simulink model "questao8_ajuste"  (R2023a)
settings: Solver=VariableStepAuto  StartTime=0.0  StopTime=160  FixedStep=1  MaxStep=0.1  RelTol=1e-3
values from neighbouring files (symbols this model uses):
  B = 0.1    [trab_controle.m]
  J = 1    [trab_controle.m]
  Km = 1/3    (= 0.333333333333)    [trab_controle.m]
  L = 0.5    [trab_controle.m]
  R = 10    [trab_controle.m]
settings Model: Creator=franz  LastModifiedBy=franz

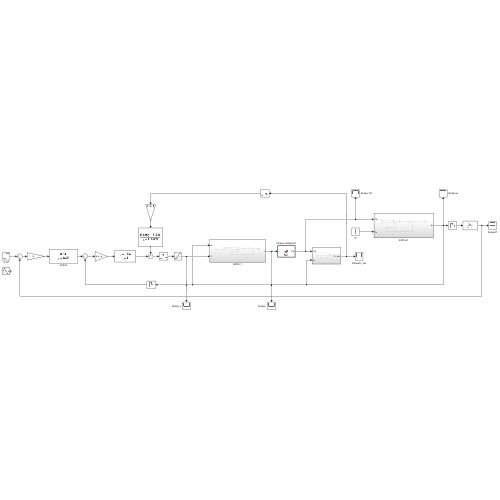
[thumbnail: Simulink's stored preview of the top-level diagram]
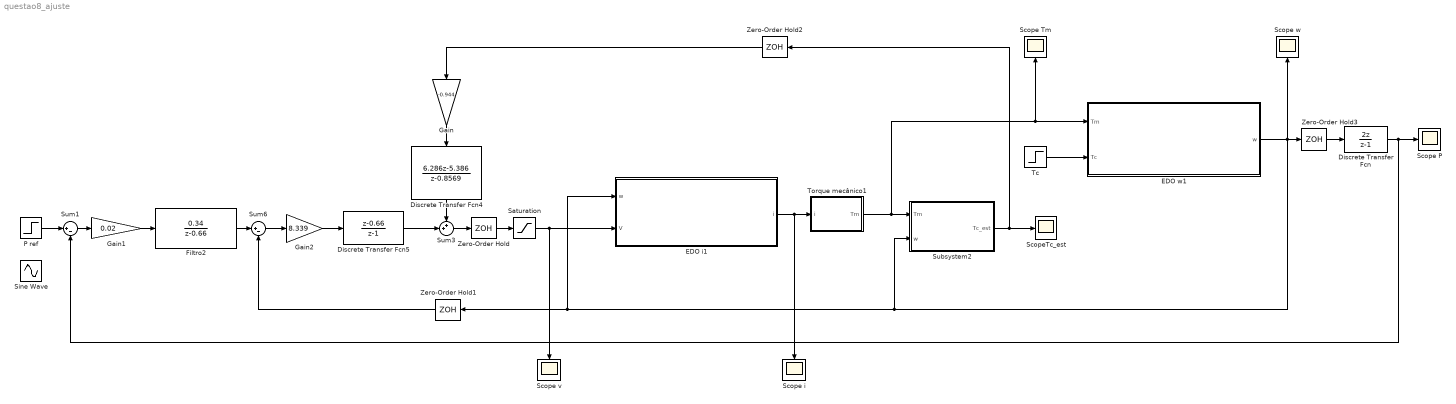
== system questao8_ajuste ==
  Discrete Transfer Fcn : DiscreteTransferFcn  Numerator=[2 0]  Denominator=[1 -1]
  Discrete Transfer Fcn4 : DiscreteTransferFcn  Numerator=[6.286 -5.386]  Denominator=[1 -0.8569]
  Discrete Transfer Fcn5 : DiscreteTransferFcn  Numerator=[1 -0.66]  Denominator=[1 -1]
  EDO i1 : Subsystem
  EDO w1 : Subsystem
  Filtro2 : DiscreteTransferFcn  Numerator=[0 0.34]  Denominator=[1 -0.66]
  Gain : Gain  Gain=-0.944
  Gain1 : Gain  Gain=0.02
  Gain2 : Gain  Gain=8.339
  P ref : Step  Time=80  After=5  SampleTime=0
  Saturation : Saturate  UpperLimit=40  LowerLimit=-40
  Scope P : Scope
  Scope Tm : Scope
  Scope i : Scope
  Scope v : Scope
  Scope w : Scope
  ScopeTc_est : Scope
  Sine Wave : Sin  Amplitude=5  Frequency=0.1  SampleTime=0
  Subsystem2 : Subsystem
  Sum1 : Sum  Inputs=|+-
  Sum3 : Sum  Inputs=++|
  Sum6 : Sum  Inputs=|+-
  Tc : Step  Time=120  Before=1.5  After=1.75  SampleTime=0
  Torque mecânico1 : MATLAB Function  TreatAsAtomicUnit=on
  Zero-Order Hold{,1..3} (4 alike) : ZeroOrderHold  SampleTime=-1
  wires:
  Discrete Transfer Fcn5/1 -> Sum3/2
  Filtro2/1 -> Sum6/1
  Discrete Transfer Fcn4/1 -> Sum3/1
  Sum6/1 -> Gain2/1
  Gain2/1 -> Discrete Transfer Fcn5/1
  Subsystem2/1(Tc_est) -> ScopeTc_est/1, Zero-Order Hold2/1
  EDO i1/1(i) -> Torque mecânico1/1(i), Scope i/1
  Torque mecânico1/1(Tm) -> Subsystem2/1(Tm), EDO w1/1(Tm), Scope Tm/1
  Tc/1 -> EDO w1/2(Tc)
  EDO w1/1(w) -> Zero-Order Hold3/1, Zero-Order Hold1/1, EDO i1/1(w), Subsystem2/2(w), Scope w/1
  Sum3/1 -> Zero-Order Hold/1
  Gain/1 -> Discrete Transfer Fcn4/1
  Zero-Order Hold/1 -> Saturation/1
  Zero-Order Hold1/1 -> Sum6/2
  Zero-Order Hold2/1 -> Gain/1
  Saturation/1 -> EDO i1/2(V), Scope v/1
  Discrete Transfer Fcn/1 -> Scope P/1, Sum1/2
  Sum1/1 -> Gain1/1
  Gain1/1 -> Filtro2/1
  Zero-Order Hold3/1 -> Discrete Transfer Fcn/1
  P ref/1 -> Sum1/1

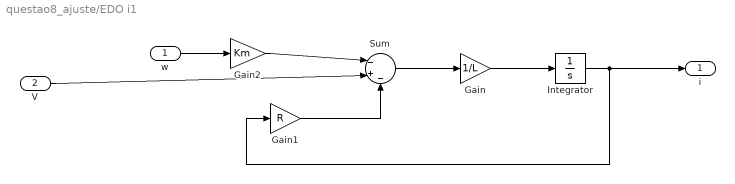
== system questao8_ajuste/EDO i1 ==
  w : Inport
  V : Inport  Port=2
  Gain : Gain  Gain=1/L
  Gain1 : Gain  Gain=R
  Gain2 : Gain  Gain=Km
  Integrator : Integrator
  Sum : Sum  Inputs=|-+-
  i : Outport
  wires:
  Gain1/1 -> Sum/3
  Integrator/1 -> i/1, Gain1/1
  Gain/1 -> Integrator/1
  Sum/1 -> Gain/1
  w/1 -> Gain2/1
  Gain2/1 -> Sum/1
  V/1 -> Sum/2

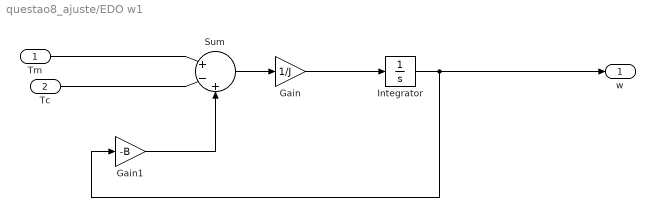
== system questao8_ajuste/EDO w1 ==
  Tm : Inport
  Tc : Inport  Port=2
  Gain : Gain  Gain=1/J
  Gain1 : Gain  Gain=-B
  Integrator : Integrator
  Sum : Sum  Inputs=|+-+
  w : Outport
  wires:
  Tm/1 -> Sum/1
  Sum/1 -> Gain/1
  Tc/1 -> Sum/2
  Gain/1 -> Integrator/1
  Gain1/1 -> Sum/3
  Integrator/1 -> Gain1/1, w/1

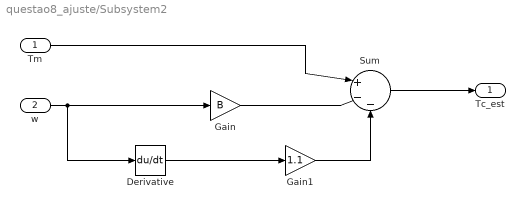
== system questao8_ajuste/Subsystem2 ==
  Tm : Inport
  w : Inport  Port=2
  Derivative : Derivative
  Gain : Gain  Gain=B
  Gain1 : Gain  Gain=1.1
  Sum : Sum  Inputs=|+--
  Tc_est : Outport
  wires:
  w/1 -> Derivative/1, Gain/1
  Gain/1 -> Sum/2
  Tm/1 -> Sum/1
  Derivative/1 -> Gain1/1
  Gain1/1 -> Sum/3
  Sum/1 -> Tc_est/1

== matlab function questao8_ajuste/Torque mecânico1 ==
  data: i input; Tm output
function Tm = fcn(i)

if i >= 0
    torque_m = 5.26*(1 - exp(-i));
else
    torque_m = -5.26*(1 - exp(i));
end
Tm = torque_m;
